simulink model "stellaris_lp_irreceive_RCA"  (R2017a)
settings: Solver=FixedStepDiscrete  StartTime=0.0  StopTime=0.5  FixedStep=ts  RelTol=1e-3  EnableMultiTasking=on
undefined symbols (not defined in the file or in its folder): ts
libraries: simulink x6, stellaris_lp_lib x4
settings Model: ExtModeTrigDuration=2  Creator=peselnikmg  LastModifiedBy=Nilim
settings DataIOCC: LimitDataPoints=on  SaveFormat=Array  SignalLoggingSaveFormat=ModelDataLogs  ReturnWorkspaceOutputs=on
settings OptimizationCC: UseDivisionForNetSlopeComputation=on  UseFloatMulNetSlope=on  UseSpecifiedMinMax=on  PassReuseOutputArgsAs=Individual arguments  ExpressionDepthLimit=2147483647  ZeroExternalMemoryAtStartup=off  ZeroInternalMemoryAtStartup=off  NoFixptDivByZeroProtection=on  EfficientFloat2IntCast=on  LifeSpan=inf  MaxStackSize=64  OptimizeBlockOrder=speed
settings DebuggingCC: ReadBeforeWriteMsg=DisableAll  WriteAfterWriteMsg=DisableAll  WriteAfterReadMsg=DisableAll  MultiTaskDSMMsg=none  IntegerOverflowMsg=error  ParameterTunabilityLossMsg=error  AssertControl=DisableAll  StateNameClashWarn=warning  NonBusSignalsTreatedAsBus=error  SFInvalidInputDataAccessInChartInitDiag=error  SFTransitionOutsideNaturalParentDiag=error  SFUnreachableExecutionPathDiag=error  SFUndirectedBroadcastEventsDiag=error  SFExecutionAtInitializationDiag=none  IntegerSaturationMsg=error
settings HardwareCC: ProdBitPerPointer=32  ProdBitPerSizeT=32  ProdBitPerPtrDiffT=32  ProdLargestAtomicInteger=Long  ProdLargestAtomicFloat=Double  ProdWordSize=32  ProdHWDeviceType=ARM Compatible->ARM Cortex
settings ModelReferenceCC: UpdateModelReferenceTargets=IfOutOfDate  PropagateSignalLabelsOutOfModel=off
settings SFSimCC: SFSimEcho=off  MATLABDynamicMemAlloc=off
settings RTWCC: SystemTargetFile=ert.tlc  HardwareBoard=Tiva TM4C123G Launchpad  TLCOptions=-aInlineSetEventsForThisBaseRateFcn=TLC_FALSE -aSuppressMultiTaskScheduler=TLC_FALSE -aRateBasedStepFcn=1  TemplateMakefile=ert_default_tmf  Description=Embedded Coder  GenerateReport=on  RTWVerbose=off  Toolchain=Texas Instruments Code Composer Studio (Tiva)  BuildConfiguration=Faster Runs  IncludeHyperlinkInReport=on  LaunchReport=on  GenerateTraceInfo=on  GenerateTraceReport=on  GenerateTraceReportSl=on  GenerateTraceReportSf=on  GenerateTraceReportEml=on
settings CodeAppCC: ForceParamTrailComments=on  IgnoreCustomStorageClasses=off  OperatorAnnotations=on  SimulinkDataObjDesc=on  SFDataObjDesc=on  MATLABFcnDesc=on  CustomSymbolStrType=$N$R$M  InsertBlockDesc=on  MATLABSourceComments=on  EnableCustomComments=on  ReqsInCode=on
settings ERTTargetCC: UtilityFuncGeneration=Shared location  CombineSignalStateStructs=on  SuppressErrorStatus=on  SupportNonFinite=off  ParenthesesLevel=Maximum  CastingMode=Standards  EnableSignedLeftShifts=off  EnableSignedRightShifts=off
settings ConfigComp: CovMetricSettings=dw  CovHtmlReporting=on  CovSaveCumulativeToWorkspaceVar=on  CovSaveSingleToWorkspaceVar=on  CovExternalEMLEnable=off

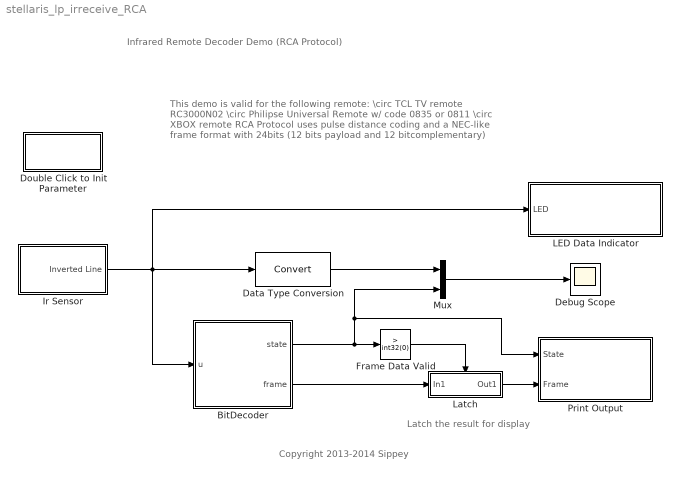
== system stellaris_lp_irreceive_RCA ==
  note: Latch the result for display
  note: This demo is valid for the following remote:
      | \circ  TCL TV remote RC3000N02
      | \circ  Philipse Universal Remote w/ code 0835 or 0811
      | \circ  XBOX remote
      |
      | RCA Protocol uses pulse distance coding and a NEC-like frame
      |  format with 24bits (12 bits payload and 12 bitcomplementary)
  note: Infrared Remote Decoder Demo (RCA Protocol)
  note: Copyright 2013-2014 Sippey
  BitDecoder : Stateflow chart  TreatAsAtomicUnit=on
  Data Type Conversion : DataTypeConversion  SampleTime=ts
  Debug Scope : Scope
  Double Click to Init Parameter : Subsystem
      settings: OpenFcn=ts=0.0001;
      mask Display: fprintf('Double-click');
  Frame Data Valid : simulink/Logic and Bit Operations/Compare To Constant  relop=>  const=int32(0)  OutDataTypeStr=boolean
  Ir Sensor : Subsystem
  LED Data Indicator : Subsystem
  Latch : Subsystem  TreatAsAtomicUnit=on
  Mux : Mux  Inputs=2
  Print Output : Subsystem
  wires:
  Mux/1 -> Debug Scope/1
  Ir Sensor/1(Inverted Line) -> BitDecoder/1(u), Data Type Conversion/1, LED Data Indicator/1(LED)
  BitDecoder/2(frame) -> Latch/1(In1)
  Latch/1(Out1) -> Print Output/2(Frame)
  Frame Data Valid/1 -> Latch/Trigger
  Data Type Conversion/1 -> Mux/1
  BitDecoder/1(state) -> Print Output/1(State), Mux/2, Frame Data Valid/1

== system stellaris_lp_irreceive_RCA/Double Click to Init Parameter ==

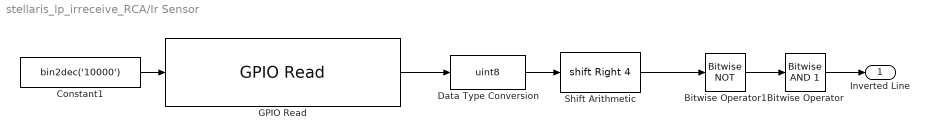
== system stellaris_lp_irreceive_RCA/Ir Sensor ==
  Bitwise Operator : simulink/Logic and Bit Operations/Bitwise Operator  logicop=AND  UseBitMask=on  BitMask=1  BitMaskRealWorld=Stored Integer
  Bitwise Operator1 : simulink/Logic and Bit Operations/Bitwise Operator  logicop=NOT  UseBitMask=off  BitMask=1  BitMaskRealWorld=Stored Integer
  Constant1 : Constant  Value=bin2dec('10000')  OutDataTypeStr=Inherit: Inherit via back propagation
  Data Type Conversion : DataTypeConversion  OutDataTypeStr=uint8  SampleTime=ts
  GPIO Read : stellaris_lp_lib/GPIO/GPIO Read  GPIO_PORTX_BASE=GPIO_PORTF_BASE  SampleTime=-1
      settings: SourceProductName=Run on Stellaris LaunchPad
  Shift Arithmetic : ArithShift  BitShiftNumber=4  BitShiftDirection=Right
  Inverted Line : Outport
  wires:
  Constant1/1 -> GPIO Read/1
  Shift Arithmetic/1 -> Bitwise Operator1/1
  GPIO Read/1 -> Data Type Conversion/1
  Bitwise Operator1/1 -> Bitwise Operator/1
  Bitwise Operator/1 -> Inverted Line/1
  Data Type Conversion/1 -> Shift Arithmetic/1

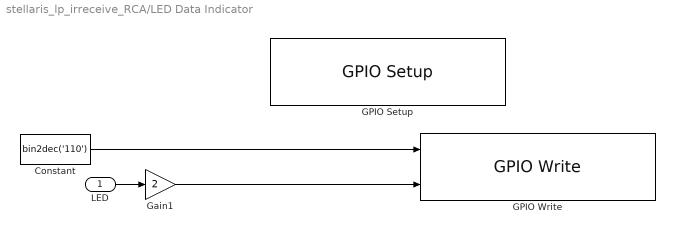
== system stellaris_lp_irreceive_RCA/LED Data Indicator ==
  LED : Inport
  Constant : Constant  Value=bin2dec('110')  OutDataTypeStr=Inherit: Inherit via back propagation
  GPIO Setup : stellaris_lp_lib/GPIO/GPIO Setup  GPIO_PORTX_BASE=GPIO_PORTF_BASE  PinsOutput_0=Input  PinsOutput_1=Output  PinsOutput_2=Output  PinsOutput_3=Output  PinsOutput_4=Input  PinsOutput_5=Input  PinsOutput_6=Input  PinsOutput_7=Input
      settings: SourceProductName=Run on Stellaris LaunchPad
  GPIO Write : stellaris_lp_lib/GPIO/GPIO Write  GPIO_PORTX_BASE=GPIO_PORTF_BASE  SampleTime=-1
      settings: SourceProductName=Run on Stellaris LaunchPad
  Gain1 : Gain  Gain=2  OutDataTypeStr=Inherit: Inherit via back propagation
  wires:
  Constant/1 -> GPIO Write/1
  Gain1/1 -> GPIO Write/2
  LED/1 -> Gain1/1

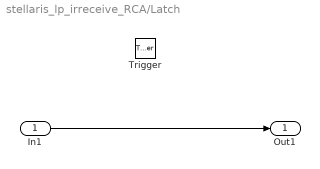
== system stellaris_lp_irreceive_RCA/Latch ==
  In1 : Inport
  Trigger : TriggerPort  VariantControl=Variant
  Out1 : Outport
  wires:
  In1/1 -> Out1/1

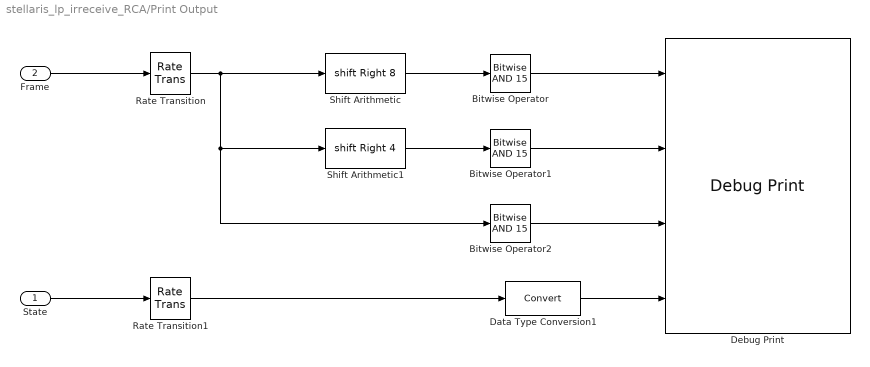
== system stellaris_lp_irreceive_RCA/Print Output ==
  State : Inport
  Frame : Inport  Port=2
  Bitwise Operator : simulink/Logic and Bit Operations/Bitwise Operator  logicop=AND  UseBitMask=on  BitMask=15  BitMaskRealWorld=Stored Integer
  Bitwise Operator1 : simulink/Logic and Bit Operations/Bitwise Operator  logicop=AND  UseBitMask=on  BitMask=15  BitMaskRealWorld=Stored Integer
  Bitwise Operator2 : simulink/Logic and Bit Operations/Bitwise Operator  logicop=AND  UseBitMask=on  BitMask=15  BitMaskRealWorld=Stored Integer
  Data Type Conversion1 : DataTypeConversion
  Debug Print : stellaris_lp_lib/Debug/Debug Print  fmt='All1: 0x%x, addr: %d, key %d, state %d'  sample_time=0.2
      settings: SourceProductName=Run on Stellaris LaunchPad
  Rate Transition : RateTransition
  Rate Transition1 : RateTransition
  Shift Arithmetic : ArithShift  BitShiftNumber=8  BitShiftDirection=Right
  Shift Arithmetic1 : ArithShift  BitShiftNumber=4  BitShiftDirection=Right
  wires:
  Shift Arithmetic/1 -> Bitwise Operator/1
  Bitwise Operator/1 -> Debug Print/1
  Shift Arithmetic1/1 -> Bitwise Operator1/1
  Rate Transition/1 -> Bitwise Operator2/1, Shift Arithmetic1/1, Shift Arithmetic/1
  Bitwise Operator1/1 -> Debug Print/2
  Bitwise Operator2/1 -> Debug Print/3
  Rate Transition1/1 -> Data Type Conversion1/1
  Frame/1 -> Rate Transition/1
  Data Type Conversion1/1 -> Debug Print/4
  State/1 -> Rate Transition1/1

== stateflow chart stellaris_lp_irreceive_RCA/BitDecoder ==
  note: Long bit ~ 2ms
      | Short bit ~1ms
      | Threshold set to 1.5ms
  note: bit timeout
  note: 4ms start pulse
      | set 3.5ms as threshold
  note: invalid start bit
  state StartSym
    state = -2;
  state BitWait
    state= -3;
  state Idle
    state = -1;
    frame=0;
  state BitDecoded
    state=-4;
  state OutStage
    state=1;
  note: output trigger
      | valid for one tick
  note: space between start bit and first data
      | pulse is 4ms and will be decoded
      | as a '1' bit, so one more bit to decode.
  BitWait -> Idle [order 4] : after(10e-3,sec)
  (default) -> Idle
  StartSym -> BitWait [order 1] : after(3.5e-3,sec)
      | [u==0]
      | {nb=0;frame=0;}
  StartSym -> Idle [order 2] : before(3.5e-3,sec)[u==0]
  BitWait -> BitDecoded [order 2] : after(1.5e-3,sec)[u==1]{frame=2*frame+1;}
  BitWait -> BitDecoded [order 3] : before(1.5e-3,sec)[u==1]{frame=2*frame;}
  Idle -> StartSym : [u==1]
  BitDecoded -> BitWait : [u==0]{nb=nb+1;}
  OutStage -> Idle
  BitWait -> OutStage [order 1] : [nb>=13]
  data: u input; state output int32 =0; nb local int32; frame output int32
